simulink model "ism"  (R2023b)
settings: Solver=VariableStepAuto  StartTime=0.0  StopTime=1  RelTol=1e-3
undefined symbols (not defined in the file): den, Ki, Kp, num
settings Model: Creator=luisf  LastModifiedBy=luisf

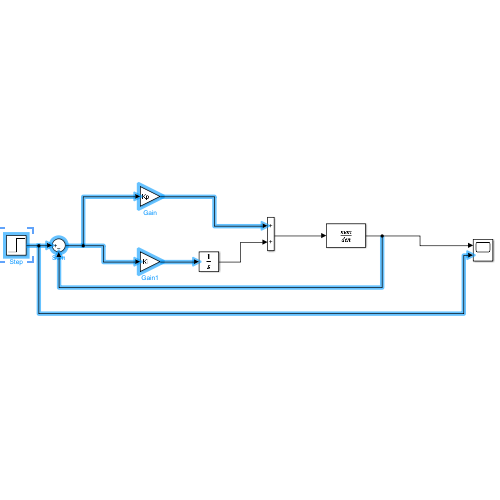
[thumbnail: Simulink's stored preview of the top-level diagram]
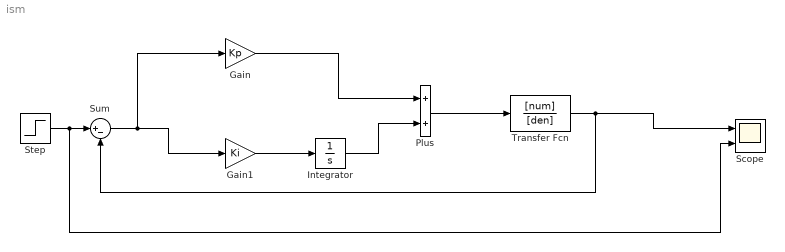
== system ism ==
  Gain : Gain  Gain=Kp
  Gain1 : Gain  Gain=Ki
  Integrator : Integrator
  Plus : Sum
  Scope : Scope  NumInputPorts=2
  Step : Step  Time=0  SampleTime=0
  Sum : Sum  Inputs=|+-
  Transfer Fcn : TransferFcn  Numerator=[num]  Denominator=[den]
  wires:
  Integrator/1 -> Plus/2
  Gain/1 -> Plus/1
  Gain1/1 -> Integrator/1
  Plus/1 -> Transfer Fcn/1
  Transfer Fcn/1 -> Sum/2, Scope/1
  Sum/1 -> Gain/1, Gain1/1
  Step/1 -> Scope/2, Sum/1
